simulink model "sensorMCUSlugsMKII_ren"  (Simulink 6.6)
settings: Solver=FixedStepDiscrete  StartTime=0.0  StopTime=10.0  FixedStep=0.01  RelTol=1e-3
InitFcn:
  | mcuInit
values from neighbouring files (symbols this model uses):
  accBiasRateLimit = 2*(.014844)/300*apSampleTime    [mcuInit.m]
  accelXCutTemp = 350.0    (= 350)    [mcuInit.m]
  axTGain1 = -0.0332796    [mcuInit.m]
  axTGain2 = 0.0543519    [mcuInit.m]
  axTMean1 = 68.41    [mcuInit.m]
  axTMean2 = 500.7    [mcuInit.m]
  barAdjust = -6    [mcuInit.m]
  baroCutoff = 0.38/(2*pi)    (= 0.0604788783749)    [mcuInit.m]
  baroCutTemp = -50.0    (= -50)    [mcuInit.m]
  baroOffset = P(2)    [mcuInit.m]
  baroScale = P(1)    [mcuInit.m]
  barTGain1 = -0.0102663    [mcuInit.m]
  barTGain2 = 0.0207608    [mcuInit.m]
  barTMean1 = -161.3    [mcuInit.m]
  barTMean2 = 347.23    [mcuInit.m]
  baseTemp = 288.215    [mcuInit.m]
  cubeAccelGain = (2.522e-3)*9.815    (= 0.02475343)    [mcuInit.m]
  cubeGyroGain = .07326*pi/180    (= 0.00127862821001)    [mcuInit.m]
  gyroBiasRateLimit = 2*(.006393)/500*apSampleTime    [mcuInit.m]
  lapseRate = -0.00198122    [mcuInit.m]
  lowRateSensorCutoff = 0.02    [mcuInit.m]
  magMeanTemp = [162.42 162.42 162.42]    [mcuInit.m]
  magOffset = 0    [mcuInit.m]
  magScale = 0.3418    [mcuInit.m]
  magTempK = [.0057 -.0423 .0426]    [mcuInit.m]
  mainSensorCutoff = 10    [mcuInit.m]
  maxDynPressure = 3000    [mcuInit.m]
  pitAdjust = -41    [mcuInit.m]
  pitCutTemp = -130.0    (= -130)    [mcuInit.m]
  pitotOffset = -1083.881038056753    (= -1083.88103806)    [mcuInit.m]
  pitotScale = 1.213292590242    (= 1.21329259024)    [mcuInit.m]
  pitTGain1 = -0.0552923    [mcuInit.m]
  pitTGain2 = -0.0950433    [mcuInit.m]
  pitTMean1 = -202.93    [mcuInit.m]
  pitTMean2 = 293.053    [mcuInit.m]
  powerOffset = P(2)    [mcuInit.m]
  powerScale = P(1)    [mcuInit.m]
  pressureSensorCutoff = 5    [mcuInit.m]
  T = 0.01    [initGPS.m]    (also in mcuInit.m)
  tempOffset = P(2)    [mcuInit.m]
  tempScale = P(1)    [mcuInit.m]
  vzCutoff = 2    [mcuInit.m]
  xCutoff = 10    [mcuInit.m]
  yCutoff = 10    [mcuInit.m]
  zCutoff = 0.2    [mcuInit.m]
undefined symbols (not defined in the file or in its folder): apSampleTime, baseHeight, DiscIntNeverNeededParam, gaind, getCubeData, getGpsMainData, getMag, GS_location, hil_getEuler, hil_getRates, hil_getRawRead, hil_getVned, hil_getXYZ, hilRead, logData, param_acc, param_mag, polesd, protParseDecode, q_quat, sensorMCUInit, spiSend, u1, u2, updateAirData, updateAttitude, updateBias, updateDiagnosticFl, updateDiagnosticSh, updateLoadData, updatePilotConsole, updatePosition, updateRawADCData, updateTimeStamp, Vb_0, y1, zerosd
libraries: dsPICdrivers x45, simulink x13, aerolibutil x4, dspmtrx3 x2, aerolibconvert2 x2
(part 3 of 4)

== system sensorMCUSlugsMKII_ren/Position and Attitude Filter/Position Filter/BlendPosVel/2 FIlter Blend ==
  HiPass : Inport
  LoPass1 : Inport  Port=2
  1D Filter : Subsystem  AncestorBlock=SLUGS_Library/Singnal Routing & Conditioning/3D Filter  RTWFcnName=TustinFilter3D  mask{zval=[0], pval=-zCutoff, kval=1, TSample=apSampleTime}
      mask prompts: zval "Zeros"; pval "Poles"; kval "Gains"; TSample "Sample Time"
      settings: RTWFcnNameOpts=User specified  RTWFileNameOpts=Use function name
      mask Display:
      | droots(zval,pval,kval)
      | port_label('input',1,'1D')
  Sum : Sum  OutDataTypeMode=single
  "Tustin Lowpass,  Auto Initial Condition4" : Subsystem  mask(Tustin1stOrderLowpassAutoInitialCondition){f=baroCutoff, T=T}
      mask prompts: f "Lowpass Frequency"; T "Sample Time"
      mask help: Takes a 3db rolloff frequency (in Hz, NOT radians/s) and a sample time. Performs a symbolic Tustin conversion and implements in a discrete filter. The initial output of the filter is set by the first sample.
      mask Help: Enter the desired 3db rolloff frequency in Hz and the sample time. Initial conditions are sampled automatically.
      mask Display: fprintf('%.2f Hz lowpass',f)
  Blend : Outport
  wires:
  HiPass/1 -> 1D Filter/1(In1)
  LoPass1/1 -> "Tustin Lowpass,  Auto Initial Condition4"/1(In1)
  1D Filter/1(Out1) -> Sum/1
  "Tustin Lowpass,  Auto Initial Condition4"/1(Out1) -> Sum/2
  Sum/1 -> Blend/1

== system sensorMCUSlugsMKII_ren/Position and Attitude Filter/Position Filter/BlendPosVel/3D Filter ==
  In1 : Inport
  Data Type Conversion1 : DataTypeConversion  OutDataTypeMode=single
  Data Type Conversion2 : DataTypeConversion  OutDataTypeMode=double
  Demux : Demux  Outputs=3
  Filter1 : Subsystem  mask(DiscretizedZeroPole){Zeros=zval, Poles=pval, Gain=kval, AbsTol=auto, SampleTime=TSample, method=tustin, Wc=1}
      mask prompts: Zeros "Zeros (enter in s-main:)"; Poles "Poles (enter in s-domain:)"; Gain "Gain (enter in s-domain:)"; AbsTol "Absolute tolerance:"; SampleTime "Sample time:"; Wc "Critical Frequency (Hz):"
      mask help: Continuous mask uses c2d to transform parameters onto the Discrete Zero-Pole block inside.
      mask init: same as sensorMCUSlugsMKII_ren/Position and Attitude Filter/Attitude Complimentary Filter COG/3D Filter/Filter1
      mask StyleString: edit,edit,edit,edit,edit,popup(zoh|foh|tustin|prewarp|matched),edit
      mask CallbackString: |||||hidecrit|
      mask Display:
      | droots(zeross,poless,gainss)
      | text( 0.5, 1.0, method, 'verticalAlignment','top')
  Filter2 : Subsystem  mask(DiscretizedZeroPole){Zeros=zval, Poles=pval, Gain=kval, AbsTol=auto, SampleTime=TSample, method=tustin, Wc=1}
      mask prompts: Zeros "Zeros (enter in s-main:)"; Poles "Poles (enter in s-domain:)"; Gain "Gain (enter in s-domain:)"; AbsTol "Absolute tolerance:"; SampleTime "Sample time:"; Wc "Critical Frequency (Hz):"
      mask help: Continuous mask uses c2d to transform parameters onto the Discrete Zero-Pole block inside.
      mask init: same as sensorMCUSlugsMKII_ren/Position and Attitude Filter/Attitude Complimentary Filter COG/3D Filter/Filter1
      mask StyleString: edit,edit,edit,edit,edit,popup(zoh|foh|tustin|prewarp|matched),edit
      mask CallbackString: |||||hidecrit|
      mask Display:
      | droots(zeross,poless,gainss)
      | text( 0.5, 1.0, method, 'verticalAlignment','top')
  Filter3 : Subsystem  mask(DiscretizedZeroPole){Zeros=zval, Poles=pval, Gain=kval, AbsTol=auto, SampleTime=TSample, method=tustin, Wc=1}
      mask prompts: Zeros "Zeros (enter in s-main:)"; Poles "Poles (enter in s-domain:)"; Gain "Gain (enter in s-domain:)"; AbsTol "Absolute tolerance:"; SampleTime "Sample time:"; Wc "Critical Frequency (Hz):"
      mask help: Continuous mask uses c2d to transform parameters onto the Discrete Zero-Pole block inside.
      mask init: same as sensorMCUSlugsMKII_ren/Position and Attitude Filter/Attitude Complimentary Filter COG/3D Filter/Filter1
      mask StyleString: edit,edit,edit,edit,edit,popup(zoh|foh|tustin|prewarp|matched),edit
      mask CallbackString: |||||hidecrit|
      mask Display:
      | droots(zeross,poless,gainss)
      | text( 0.5, 1.0, method, 'verticalAlignment','top')
  myMux Fun1 : Stateflow chart
  Out1 : Outport
  wires:
  myMux Fun1/1(y) -> Data Type Conversion1/1
  In1/1 -> Data Type Conversion2/1
  Filter3/1(Out1) -> myMux Fun1/3(u3)
  Filter2/1(Out1) -> myMux Fun1/2(u2)
  Filter1/1(Out1) -> myMux Fun1/1(u1)
  Demux/3 -> Filter3/1(In1)
  Demux/2 -> Filter2/1(In1)
  Demux/1 -> Filter1/1(In1)
  Data Type Conversion2/1 -> Demux/1
  Data Type Conversion1/1 -> Out1/1

== system sensorMCUSlugsMKII_ren/Position and Attitude Filter/Position Filter/BlendPosVel/CompFiltRate ==
  Rate : Inport
  LoPass : Inport  Port=2
  1D Filter1 : Subsystem  AncestorBlock=SLUGS_Library/Singnal Routing & Conditioning/3D Filter  RTWFcnName=TustinFilter3D  mask{zval=[], pval=[0], kval=1, TSample=T}
      mask prompts: zval "Zeros"; pval "Poles"; kval "Gains"; TSample "Sample Time"
      settings: RTWFcnNameOpts=User specified  RTWFileNameOpts=Use function name
      mask Display:
      | droots(zval,pval,kval)
      | port_label('input',1,'1D')
  Gain : Gain  Gain=omega
  Sum : Sum  Inputs=++|
  Sum1 : Sum  Inputs=|+-
  Unit Delay : UnitDelay  Orientation=left  SampleTime=T
  Blend : Outport
  wires:
  Unit Delay/1 -> Sum1/2
  LoPass/1 -> Sum1/1
  Sum1/1 -> Gain/1
  Gain/1 -> Sum/2
  Rate/1 -> Sum/1
  Sum/1 -> 1D Filter1/1(In1)
  1D Filter1/1(Out1) -> Unit Delay/1, Blend/1

== system sensorMCUSlugsMKII_ren/Position and Attitude Filter/Position Filter/BlendPosVel/CompFiltRate1 ==
  Rate : Inport
  LoPass : Inport  Port=2
  1D Filter1 : Subsystem  AncestorBlock=SLUGS_Library/Singnal Routing & Conditioning/3D Filter  RTWFcnName=TustinFilter3D  mask{zval=[], pval=[0], kval=1, TSample=T}
      mask prompts: zval "Zeros"; pval "Poles"; kval "Gains"; TSample "Sample Time"
      settings: RTWFcnNameOpts=User specified  RTWFileNameOpts=Use function name
      mask Display:
      | droots(zval,pval,kval)
      | port_label('input',1,'1D')
  Gain : Gain  Gain=omega
  Sum : Sum  Inputs=++|
  Sum1 : Sum  Inputs=|+-
  Unit Delay : UnitDelay  Orientation=left  SampleTime=T
  Blend : Outport
  wires:
  Unit Delay/1 -> Sum1/2
  LoPass/1 -> Sum1/1
  Sum1/1 -> Gain/1
  Gain/1 -> Sum/2
  Rate/1 -> Sum/1
  Sum/1 -> 1D Filter1/1(In1)
  1D Filter1/1(Out1) -> Unit Delay/1, Blend/1

== system sensorMCUSlugsMKII_ren/Position and Attitude Filter/Position Filter/BlendPosVel/CompRateOnly ==
  LoPass : Inport
  1D Filter1 : Subsystem  AncestorBlock=SLUGS_Library/Singnal Routing & Conditioning/3D Filter  RTWFcnName=TustinFilter3D  mask{zval=[], pval=[0], kval=1, TSample=T}
      mask prompts: zval "Zeros"; pval "Poles"; kval "Gains"; TSample "Sample Time"
      settings: RTWFcnNameOpts=User specified  RTWFileNameOpts=Use function name
      mask Display:
      | droots(zval,pval,kval)
      | port_label('input',1,'1D')
  Gain : Gain  Gain=omega
  Sum1 : Sum  Inputs=|+-
  Unit Delay : UnitDelay  Orientation=left  SampleTime=T
  Rate_hat : Outport
  wires:
  Unit Delay/1 -> Sum1/2
  LoPass/1 -> Sum1/1
  Sum1/1 -> Gain/1
  Gain/1 -> Rate_hat/1, 1D Filter1/1(In1)
  1D Filter1/1(Out1) -> Unit Delay/1

== system sensorMCUSlugsMKII_ren/Position and Attitude Filter/Position Filter/BlendPosVel/Subsystem ==
  Vn : Inport
  Ve : Inport  Port=2
  New GPS : Inport  Orientation=up  Port=3
  Enable : EnablePort
  Embedded MATLAB Function : Stateflow chart
  Embedded MATLAB Function1 : Stateflow chart
  Vn_fil : Outport  OutputWhenDisabled=reset  InitialOutput=0
  Ve_fil : Outport  Port=2  OutputWhenDisabled=reset  InitialOutput=0
  wires:
  New GPS/1 -> Embedded MATLAB Function1/2(NewGPS), Embedded MATLAB Function/2(NewGPS)
  Vn/1 -> Embedded MATLAB Function/1(u)
  Ve/1 -> Embedded MATLAB Function1/1(u)
  Embedded MATLAB Function/1(y) -> Vn_fil/1
  Embedded MATLAB Function1/1(y) -> Ve_fil/1

== system sensorMCUSlugsMKII_ren/Sensor Data/Sensor Suite/Cube Signal Cond1/3D Tustin Lowpass, Auto Initial Condition ==
  In1 : Inport
  Constant : Constant  Value=T
  Constant1 : Constant  Value=f
  Constant2 : Constant  Value=T
  Constant3 : Constant  Value=f
  Constant4 : Constant  Value=T
  Constant5 : Constant  Value=f
  Demux : Demux  Outputs=3
  Embedded MATLAB Function : Stateflow chart
  Embedded MATLAB Function1 : Stateflow chart
  Embedded MATLAB Function2 : Stateflow chart
  myMux Fun : Stateflow chart
  Out1 : Outport
  wires:
  myMux Fun/1(y) -> Out1/1
  In1/1 -> Demux/1
  Embedded MATLAB Function1/1(y) -> myMux Fun/2(u2)
  Demux/3 -> Embedded MATLAB Function2/1(u)
  Demux/2 -> Embedded MATLAB Function1/1(u)
  Demux/1 -> Embedded MATLAB Function/1(u)
  Embedded MATLAB Function2/1(y) -> myMux Fun/3(u3)
  Constant5/1 -> Embedded MATLAB Function2/3(f)
  Constant4/1 -> Embedded MATLAB Function2/2(T)
  Constant3/1 -> Embedded MATLAB Function1/3(f)
  Constant2/1 -> Embedded MATLAB Function1/2(T)
  Embedded MATLAB Function/1(y) -> myMux Fun/1(u1)
  Constant1/1 -> Embedded MATLAB Function/3(f)
  Constant/1 -> Embedded MATLAB Function/2(T)

== system sensorMCUSlugsMKII_ren/Sensor Data/Sensor Suite/Cube Signal Cond1/3D Tustin Lowpass, Auto Initial Condition1 ==
  In1 : Inport
  Constant : Constant  Value=T
  Constant1 : Constant  Value=f
  Constant2 : Constant  Value=T
  Constant3 : Constant  Value=f
  Constant4 : Constant  Value=T
  Constant5 : Constant  Value=f
  Demux : Demux  Outputs=3
  Embedded MATLAB Function : Stateflow chart
  Embedded MATLAB Function1 : Stateflow chart
  Embedded MATLAB Function2 : Stateflow chart
  myMux Fun : Stateflow chart
  Out1 : Outport
  wires:
  myMux Fun/1(y) -> Out1/1
  In1/1 -> Demux/1
  Embedded MATLAB Function1/1(y) -> myMux Fun/2(u2)
  Demux/3 -> Embedded MATLAB Function2/1(u)
  Demux/2 -> Embedded MATLAB Function1/1(u)
  Demux/1 -> Embedded MATLAB Function/1(u)
  Embedded MATLAB Function2/1(y) -> myMux Fun/3(u3)
  Constant5/1 -> Embedded MATLAB Function2/3(f)
  Constant4/1 -> Embedded MATLAB Function2/2(T)
  Constant3/1 -> Embedded MATLAB Function1/3(f)
  Constant2/1 -> Embedded MATLAB Function1/2(T)
  Embedded MATLAB Function/1(y) -> myMux Fun/1(u1)
  Constant1/1 -> Embedded MATLAB Function/3(f)
  Constant/1 -> Embedded MATLAB Function/2(T)

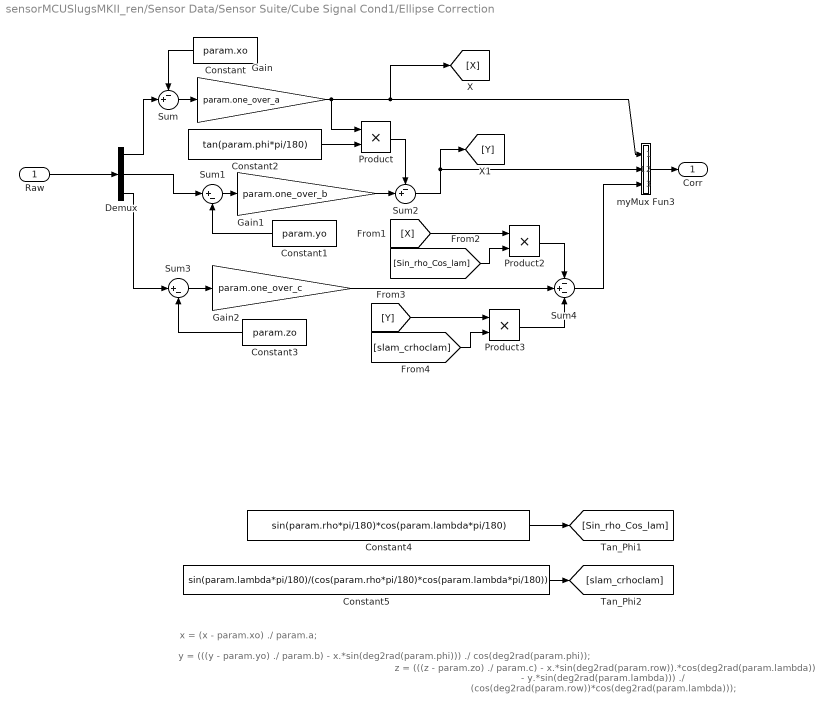
== system sensorMCUSlugsMKII_ren/Sensor Data/Sensor Suite/Cube Signal Cond1/Ellipse Correction ==
  note: x = (x - param.xo) ./ param.a;
  note: y = (((y - param.yo) ./ param.b) - x.*sin(deg2rad(param.phi))) ./ cos(deg2rad(param.phi));
  note: z = (((z - param.zo) ./ param.c) - x.*sin(deg2rad(param.row)).*cos(deg2rad(param.lambda)) - y.*sin(deg2rad(param.lambda))) ./ (cos(deg2rad(param.row))*cos(deg2rad(param.lambda)));
  Raw : Inport
  Constant : Constant  Orientation=left  Value=param.xo  OutDataTypeMode=single
  Constant1 : Constant  Orientation=left  Value=param.yo  OutDataTypeMode=single
  Constant2 : Constant  Value=tan(param.phi*pi/180)  OutDataTypeMode=single
  Constant3 : Constant  Orientation=left  Value=param.zo  OutDataTypeMode=single
  Constant4 : Constant  Value=sin(param.rho*pi/180)*cos(param.lambda*pi/180)  OutDataTypeMode=single
  Constant5 : Constant  Value=sin(param.lambda*pi/180)/(cos(param.rho*pi/180)*cos(param.lambda*pi/180))  VectorParams1D=off  OutDataTypeMode=single
  Demux : Demux  Outputs=3
  Gain : Gain  Gain=param.one_over_a
  Gain1 : Gain  Gain=param.one_over_b
  Gain2 : Gain  Gain=param.one_over_c
  Product : Product  RndMeth=Zero
  Product2 : Product  RndMeth=Zero
  Product3 : Product  RndMeth=Zero
  Sum : Sum  Inputs=-+|
  Sum1 : Sum  Inputs=|+-
  Sum2 : Sum  Inputs=-+|
  Sum3 : Sum  Inputs=|+-
  Sum4 : Sum  Inputs=-+-
  myMux Fun3 : Stateflow chart  AncestorBlock=SLUGS_Library/Singnal Routing & Conditioning/myMux Fun3
  Corr : Outport
  wires:
  Raw/1 -> Demux/1
  Demux/1 -> Sum/2
  Constant/1 -> Sum/1
  Sum/1 -> Gain/1
  Gain/1 -> [X], Product/1, myMux Fun3/1(u1)
  Sum1/1 -> Gain1/1
  myMux Fun3/1(y) -> Corr/1
  Constant1/1 -> Sum1/2
  Demux/2 -> Sum1/1
  Constant2/1 -> Product/2
  Gain1/1 -> Sum2/2
  Product/1 -> Sum2/1
  Sum2/1 -> [Y], myMux Fun3/2(u2)
  Sum3/1 -> Gain2/1
  Constant3/1 -> Sum3/2
  Gain2/1 -> Sum4/2
  Demux/3 -> Sum3/1
  [X] -> Product2/1
  [Sin_rho_Cos_lam] -> Product2/2
  Product2/1 -> Sum4/1
  [Y] -> Product3/1
  [slam_crhoclam] -> Product3/2
  Product3/1 -> Sum4/3
  Sum4/1 -> myMux Fun3/3(u3)
  Constant4/1 -> [Sin_rho_Cos_lam]
  Constant5/1 -> [slam_crhoclam]

== system sensorMCUSlugsMKII_ren/Sensor Data/Sensor Suite/Cube Signal Cond1/Rotate Cube Axis ==
  Raw : Inport
  Selector : Selector  IndexOptions=Index vector (dialog)  Indices=[2 1 3]  OutputSizes=1  InputPortWidth=3
  "[ -1 -1 -1]" : Gain  Gain=[-1 -1 -1]
  Rotated : Outport
  wires:
  Selector/1 -> "[ -1 -1 -1]"/1
  Raw/1 -> Selector/1
  "[ -1 -1 -1]"/1 -> Rotated/1

== system sensorMCUSlugsMKII_ren/Sensor Data/Sensor Suite/Cube Signal Cond1/Rotate Cube Axis  ==
  Raw : Inport
  Selector : Selector  IndexOptions=Index vector (dialog)  Indices=[2 1 3]  OutputSizes=1  InputPortWidth=3
  Rotated : Outport
  wires:
  Raw/1 -> Selector/1
  Selector/1 -> Rotated/1

== system sensorMCUSlugsMKII_ren/Sensor Data/Sensor Suite/Cube Signal Cond1/Temp Compensate Accel X ==
  Temp : Inport
  Accel X : Inport  Port=2
  Compare To Constant : simulink/Logic and Bit Operations/Compare To Constant  SystemSampleTime=-1  relop=<  const=accelXCutTemp  LogicOutDataTypeMode=uint8  ZeroCross=off
  Hi Temp Compensation : Subsystem  mask{alpha=axTGain2, tempMean=axTMean2}
      mask prompts: alpha "Tempearature Coeficient (K_t)"; tempMean "Calibration Temperature Mean (T_avg)"
      mask help:
      | This block implements a temperature compensation. It implmements the following equation:
      |
      | M_tc = M_raw - K_t(T - T_avg)
  Lo Temp Compensation : Subsystem  mask{alpha=axTGain1, tempMean=axTMean1}
      mask prompts: alpha "Tempearature Coeficient (K_t)"; tempMean "Calibration Temperature Mean (T_avg)"
      mask help:
      | This block implements a temperature compensation. It implmements the following equation:
      |
      | M_tc = M_raw - K_t(T - T_avg)
  Logical Operator : Logic  Operator=NOT  AllPortsSameDT=off  OutDataTypeMode=Boolean
  Merge : Merge
  "Tustin Lowpass, Auto Initial Condition1" : Subsystem  mask(Tustin1stOrderLowpassAutoInitialCondition){f=1, T=T}
      mask prompts: f "Lowpass Frequency"; T "Sample Time"
      mask help: Takes a 3db rolloff frequency (in Hz, NOT radians/s) and a sample time. Performs a symbolic Tustin conversion and implements in a discrete filter. The initial output of the filter is set by the first sample.
      mask Help: Enter the desired 3db rolloff frequency in Hz and the sample time. Initial conditions are sampled automatically.
      mask Display: fprintf('%.2f Hz lowpass',f)
  Accel X_c : Outport
  wires:
  "Tustin Lowpass, Auto Initial Condition1"/1(Out1) -> Accel X_c/1
  Compare To Constant/1 -> Logical Operator/1, Lo Temp Compensation/Enable
  Temp/1 -> Compare To Constant/1, Hi Temp Compensation/2(Temp Raw), Lo Temp Compensation/2(Temp Raw)
  Accel X/1 -> Hi Temp Compensation/1(Raw), Lo Temp Compensation/1(Raw)
  Hi Temp Compensation/1(Comp) -> Merge/1
  Lo Temp Compensation/1(Comp) -> Merge/2
  Merge/1 -> "Tustin Lowpass, Auto Initial Condition1"/1(In1)
  Logical Operator/1 -> Hi Temp Compensation/Enable

== system sensorMCUSlugsMKII_ren/Sensor Data/Sensor Suite/Low Pass Filtering,Temperature Compensation and Calibration1/3D Tustin Lowpass, Auto Initial Condition ==
  In1 : Inport
  Constant : Constant  Value=T
  Constant1 : Constant  Value=f
  Constant2 : Constant  Value=T
  Constant3 : Constant  Value=f
  Constant4 : Constant  Value=T
  Constant5 : Constant  Value=f
  Demux : Demux  Outputs=3
  Embedded MATLAB Function : Stateflow chart
  Embedded MATLAB Function1 : Stateflow chart
  Embedded MATLAB Function2 : Stateflow chart
  myMux Fun : Stateflow chart
  Out1 : Outport
  wires:
  myMux Fun/1(y) -> Out1/1
  In1/1 -> Demux/1
  Embedded MATLAB Function1/1(y) -> myMux Fun/2(u2)
  Demux/3 -> Embedded MATLAB Function2/1(u)
  Demux/2 -> Embedded MATLAB Function1/1(u)
  Demux/1 -> Embedded MATLAB Function/1(u)
  Embedded MATLAB Function2/1(y) -> myMux Fun/3(u3)
  Constant5/1 -> Embedded MATLAB Function2/3(f)
  Constant4/1 -> Embedded MATLAB Function2/2(T)
  Constant3/1 -> Embedded MATLAB Function1/3(f)
  Constant2/1 -> Embedded MATLAB Function1/2(T)
  Embedded MATLAB Function/1(y) -> myMux Fun/1(u1)
  Constant1/1 -> Embedded MATLAB Function/3(f)
  Constant/1 -> Embedded MATLAB Function/2(T)

== system sensorMCUSlugsMKII_ren/Sensor Data/Sensor Suite/Low Pass Filtering,Temperature Compensation and Calibration1/Baro Altimeter ==
  Static (Pa) : Inport  Orientation=up
  Compute Barometric Height : Subsystem  mask{baseTemp=baseTemp, LapseRate=lapseRate}
      mask prompts: baseTemp "Base Station Temperature (K)"; LapseRate "Lapse Rate (C/ft)"
      mask help:
      | Produces Altitude in meters from Barometric Pressure in Pascals. Altitude is valid from MSL to 6000 ft.
      |
      | The method implemented here was developed by Ren Curry
  Constant1 : Constant  Value=baseHeight  OutDataTypeMode=single
  Enabled Subsystem : Subsystem  TreatAsAtomicUnit=on
  Enables/Disables the Computation of  initial Baro Bias : Stateflow chart
  Initial Baro Bias : Subsystem  TreatAsAtomicUnit=on
  Logical Operator : Logic  Orientation=down  Operator=NOT  AllPortsSameDT=off  OutDataTypeMode=Boolean
  Sum1 : Sum  Inputs=++|  OutDataTypeMode=single
  Zero Out Height : Subsystem  TreatAsAtomicUnit=on
  Altitude : Outport
  wires:
  Compute Barometric Height/1("Altitude, m") -> Zero Out Height/2(Computed Height), Sum1/2
  Static (Pa)/1 -> Initial Baro Bias/1(Baro (Pa)), Compute Barometric Height/3(Baro (Pa))
  Enables/Disables the Computation of  initial Baro Bias/1(tOut) -> Initial Baro Bias/Enable, Zero Out Height/Enable, Logical Operator/1
  Constant1/1 -> Compute Barometric Height/1(Base Height (m)), Zero Out Height/1(Base Height)
  Initial Baro Bias/1(Baro (Gnd)) -> Compute Barometric Height/2(Base Pressure (Pa))
  Zero Out Height/1(Height Offset) -> Sum1/1
  Logical Operator/1 -> Enabled Subsystem/Enable
  Sum1/1 -> Enabled Subsystem/1(In1)
  Enabled Subsystem/1(Out1) -> Altitude/1

== system sensorMCUSlugsMKII_ren/Sensor Data/Sensor Suite/Low Pass Filtering,Temperature Compensation and Calibration1/Barometer Unit Conversion ==
  Raw : Inport
  Bias : Constant  Value=bias  OutDataTypeMode=single
  Divide : Product  OutDataTypeMode=single  OutScaling=2^-10
  Gains : Constant  Value=gains  OutDataTypeMode=single
  Sum : Sum  Inputs=|++  OutDataTypeMode=single
  Comp : Outport
  wires:
  Bias/1 -> Sum/2
  Raw/1 -> Divide/2
  Gains/1 -> Divide/1
  Divide/1 -> Sum/1
  Sum/1 -> Comp/1

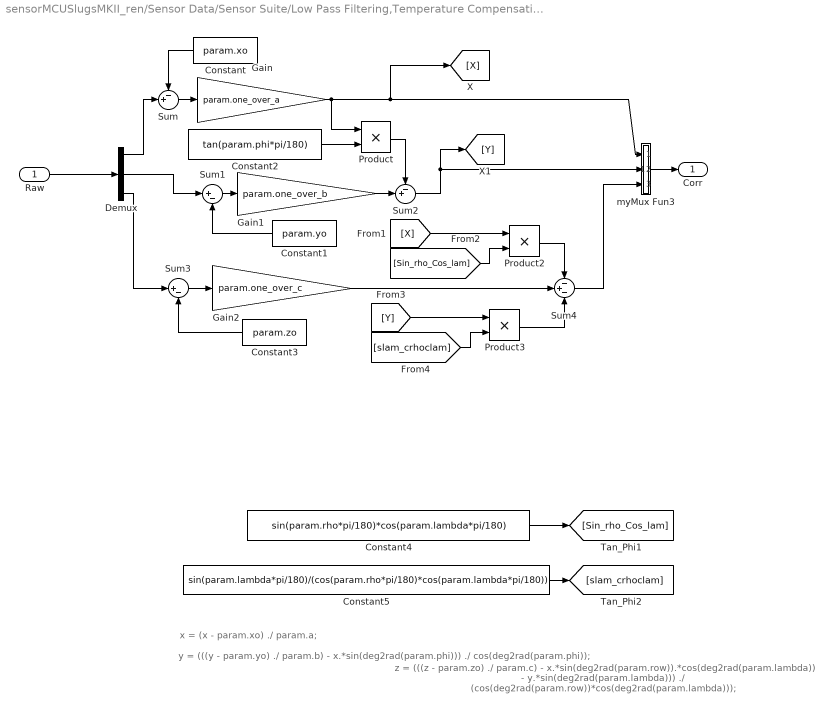
== system sensorMCUSlugsMKII_ren/Sensor Data/Sensor Suite/Low Pass Filtering,Temperature Compensation and Calibration1/Ellipse Correction ==
  note: x = (x - param.xo) ./ param.a;
  note: y = (((y - param.yo) ./ param.b) - x.*sin(deg2rad(param.phi))) ./ cos(deg2rad(param.phi));
  note: z = (((z - param.zo) ./ param.c) - x.*sin(deg2rad(param.row)).*cos(deg2rad(param.lambda)) - y.*sin(deg2rad(param.lambda))) ./ (cos(deg2rad(param.row))*cos(deg2rad(param.lambda)));
  Raw : Inport
  Constant : Constant  Orientation=left  Value=param.xo  OutDataTypeMode=single
  Constant1 : Constant  Orientation=left  Value=param.yo  OutDataTypeMode=single
  Constant2 : Constant  Value=tan(param.phi*pi/180)  OutDataTypeMode=single
  Constant3 : Constant  Orientation=left  Value=param.zo  OutDataTypeMode=single
  Constant4 : Constant  Value=sin(param.rho*pi/180)*cos(param.lambda*pi/180)  OutDataTypeMode=single
  Constant5 : Constant  Value=sin(param.lambda*pi/180)/(cos(param.rho*pi/180)*cos(param.lambda*pi/180))  VectorParams1D=off  OutDataTypeMode=single
  Demux : Demux  Outputs=3
  Gain : Gain  Gain=param.one_over_a
  Gain1 : Gain  Gain=param.one_over_b
  Gain2 : Gain  Gain=param.one_over_c
  Product : Product  RndMeth=Zero
  Product2 : Product  RndMeth=Zero
  Product3 : Product  RndMeth=Zero
  Sum : Sum  Inputs=-+|
  Sum1 : Sum  Inputs=|+-
  Sum2 : Sum  Inputs=-+|
  Sum3 : Sum  Inputs=|+-
  Sum4 : Sum  Inputs=-+-
  myMux Fun3 : Stateflow chart  AncestorBlock=SLUGS_Library/Singnal Routing & Conditioning/myMux Fun3
  Corr : Outport
  wires:
  Raw/1 -> Demux/1
  Demux/1 -> Sum/2
  Constant/1 -> Sum/1
  Sum/1 -> Gain/1
  Gain/1 -> [X], Product/1, myMux Fun3/1(u1)
  Sum1/1 -> Gain1/1
  myMux Fun3/1(y) -> Corr/1
  Constant1/1 -> Sum1/2
  Demux/2 -> Sum1/1
  Constant2/1 -> Product/2
  Gain1/1 -> Sum2/2
  Product/1 -> Sum2/1
  Sum2/1 -> [Y], myMux Fun3/2(u2)
  Sum3/1 -> Gain2/1
  Constant3/1 -> Sum3/2
  Gain2/1 -> Sum4/2
  Demux/3 -> Sum3/1
  [X] -> Product2/1
  [Sin_rho_Cos_lam] -> Product2/2
  Product2/1 -> Sum4/1
  [Y] -> Product3/1
  [slam_crhoclam] -> Product3/2
  Product3/1 -> Sum4/3
  Sum4/1 -> myMux Fun3/3(u3)
  Constant4/1 -> [Sin_rho_Cos_lam]
  Constant5/1 -> [slam_crhoclam]

== system sensorMCUSlugsMKII_ren/Sensor Data/Sensor Suite/Low Pass Filtering,Temperature Compensation and Calibration1/Magnetometer Unit Conversion ==
  Raw : Inport
  Bias : Constant  Value=bias  OutDataTypeMode=single
  Divide : Product  OutDataTypeMode=single  OutScaling=2^-10
  Gains : Constant  Value=gains  OutDataTypeMode=single
  Sum : Sum  Inputs=|++  OutDataTypeMode=single
  Comp : Outport
  wires:
  Bias/1 -> Sum/2
  Raw/1 -> Divide/2
  Gains/1 -> Divide/1
  Divide/1 -> Sum/1
  Sum/1 -> Comp/1

== system sensorMCUSlugsMKII_ren/Sensor Data/Sensor Suite/Low Pass Filtering,Temperature Compensation and Calibration1/Magnetometers Temp Compensation ==
  Raw : Inport
  Temp Raw : Inport  Port=2
  Divide1 : Product  OutDataTypeMode=single  OutScaling=2^-10
  Mean Temperature for Calibration : Constant  Value=tempMean  OutDataTypeMode=single
  Sum1 : Sum  Inputs=|+-  OutDataTypeMode=single
  Sum2 : Sum  Inputs=|+-  OutDataTypeMode=single
  gains : Constant  Value=alpha  OutDataTypeMode=single
  Comp : Outport
  wires:
  Sum2/1 -> Comp/1
  Divide1/1 -> Sum2/2
  gains/1 -> Divide1/1
  Sum1/1 -> Divide1/2
  Temp Raw/1 -> Sum1/1
  Raw/1 -> Sum2/1
  Mean Temperature for Calibration/1 -> Sum1/2

== system sensorMCUSlugsMKII_ren/Sensor Data/Sensor Suite/Low Pass Filtering,Temperature Compensation and Calibration1/Pitot Unit Conversion ==
  Raw : Inport
  Bias : Constant  Value=bias  OutDataTypeMode=single
  Divide : Product  OutDataTypeMode=single  OutScaling=2^-10
  Gains : Constant  Value=gains  OutDataTypeMode=single
  Sum : Sum  Inputs=|++  OutDataTypeMode=single
  Comp : Outport
  wires:
  Bias/1 -> Sum/2
  Raw/1 -> Divide/2
  Gains/1 -> Divide/1
  Divide/1 -> Sum/1
  Sum/1 -> Comp/1

== system sensorMCUSlugsMKII_ren/Sensor Data/Sensor Suite/Low Pass Filtering,Temperature Compensation and Calibration1/Power Unit Conversion ==
  Raw : Inport
  Bias : Constant  Value=bias  OutDataTypeMode=single
  Divide : Product  OutDataTypeMode=single  OutScaling=2^-10
  Gains : Constant  Value=gains  OutDataTypeMode=single
  Sum : Sum  Inputs=|++  OutDataTypeMode=single
  Comp : Outport
  wires:
  Bias/1 -> Sum/2
  Raw/1 -> Divide/2
  Gains/1 -> Divide/1
  Divide/1 -> Sum/1
  Sum/1 -> Comp/1

== system sensorMCUSlugsMKII_ren/Sensor Data/Sensor Suite/Low Pass Filtering,Temperature Compensation and Calibration1/Rotate Mags Axis ==
  Raw : Inport
  Selector : Selector  IndexOptions=Index vector (dialog)  Indices=[2 1 3]  OutputSizes=1  InputPortWidth=3
  "[ 1 -1 1]" : Gain  Gain=[-1 -1 1]
  Rotated : Outport
  wires:
  Selector/1 -> "[ 1 -1 1]"/1
  Raw/1 -> Selector/1
  "[ 1 -1 1]"/1 -> Rotated/1

== system sensorMCUSlugsMKII_ren/Sensor Data/Sensor Suite/Low Pass Filtering,Temperature Compensation and Calibration1/Temp Compensate Accel X1 ==
  Temp : Inport
  Dynamic : Inport  Port=2
  Compare To Constant : simulink/Logic and Bit Operations/Compare To Constant  SystemSampleTime=-1  relop=<  const=pitCutTemp  LogicOutDataTypeMode=uint8  ZeroCross=off
  Display : Display
  Display2 : Display
  Hi Temp Compensation2 : Subsystem  mask{alpha=pitTGain2, tempMean=pitTMean2}
      mask prompts: alpha "Tempearature Coeficient (K_t)"; tempMean "Calibration Temperature Mean (T_avg)"
      mask help:
      | This block implements a temperature compensation. It implmements the following equation:
      |
      | M_tc = M_raw - K_t(T - T_avg)
  Lo Temp Compensation : Subsystem  mask{alpha=pitTGain1, tempMean=pitTMean1}
      mask prompts: alpha "Tempearature Coeficient (K_t)"; tempMean "Calibration Temperature Mean (T_avg)"
      mask help:
      | This block implements a temperature compensation. It implmements the following equation:
      |
      | M_tc = M_raw - K_t(T - T_avg)
  Logical Operator : Logic  Operator=NOT  AllPortsSameDT=off  OutDataTypeMode=Boolean
  Merge : Merge
  Baro_c : Outport
  wires:
  Hi Temp Compensation2/1(Comp) -> Merge/1
  Logical Operator/1 -> Hi Temp Compensation2/Enable, Display2/1
  Merge/1 -> Baro_c/1, Display/1
  Dynamic/1 -> Lo Temp Compensation/1(Raw), Hi Temp Compensation2/1(Raw)
  Temp/1 -> Compare To Constant/1, Lo Temp Compensation/2(Temp Raw), Hi Temp Compensation2/2(Temp Raw)
  Compare To Constant/1 -> Lo Temp Compensation/Enable, Logical Operator/1
  Lo Temp Compensation/1(Comp) -> Merge/2

== system sensorMCUSlugsMKII_ren/Sensor Data/Sensor Suite/Low Pass Filtering,Temperature Compensation and Calibration1/Temp Compensate Baro ==
  Temp : Inport
  Baro : Inport  Port=2
  Compare To Constant : simulink/Logic and Bit Operations/Compare To Constant  SystemSampleTime=-1  relop=<  const=baroCutTemp  LogicOutDataTypeMode=uint8  ZeroCross=off
  Hi Temp Compensation : Subsystem  mask{alpha=barTGain2, tempMean=barTMean2}
      mask prompts: alpha "Tempearature Coeficient (K_t)"; tempMean "Calibration Temperature Mean (T_avg)"
      mask help:
      | This block implements a temperature compensation. It implmements the following equation:
      |
      | M_tc = M_raw - K_t(T - T_avg)
  Lo Temp Compensation : Subsystem  mask{alpha=barTGain1, tempMean=barTMean1}
      mask prompts: alpha "Tempearature Coeficient (K_t)"; tempMean "Calibration Temperature Mean (T_avg)"
      mask help:
      | This block implements a temperature compensation. It implmements the following equation:
      |
      | M_tc = M_raw - K_t(T - T_avg)
  Logical Operator : Logic  Operator=NOT  AllPortsSameDT=off  OutDataTypeMode=Boolean
  Merge : Merge
  Baro_c : Outport
  wires:
  Compare To Constant/1 -> Logical Operator/1, Lo Temp Compensation/Enable
  Temp/1 -> Compare To Constant/1, Hi Temp Compensation/2(Temp Raw), Lo Temp Compensation/2(Temp Raw)
  Baro/1 -> Hi Temp Compensation/1(Raw), Lo Temp Compensation/1(Raw)
  Lo Temp Compensation/1(Comp) -> Merge/2
  Merge/1 -> Baro_c/1
  Logical Operator/1 -> Hi Temp Compensation/Enable
  Hi Temp Compensation/1(Comp) -> Merge/1

== system sensorMCUSlugsMKII_ren/Sensor Data/Sensor Suite/Low Pass Filtering,Temperature Compensation and Calibration1/Thermistor Unit Conversion ==
  Raw : Inport
  Bias : Constant  Value=bias  OutDataTypeMode=single
  Divide : Product  OutDataTypeMode=single  OutScaling=2^-10
  Gains : Constant  Value=gains  OutDataTypeMode=single
  Sum : Sum  Inputs=|++  OutDataTypeMode=single
  Comp : Outport
  wires:
  Sum/1 -> Comp/1
  Divide/1 -> Sum/1
  Gains/1 -> Divide/1
  Raw/1 -> Divide/2
  Bias/1 -> Sum/2

== system sensorMCUSlugsMKII_ren/Sensor Data/Sensor Suite/Low Pass Filtering,Temperature Compensation and Calibration1/Tustin Lowpass, Auto Initial Condition1 ==
  In1 : Inport
  Constant : Constant  Value=T
  Constant1 : Constant  Value=f
  Embedded MATLAB Function : Stateflow chart
  Out1 : Outport
  wires:
  Constant/1 -> Embedded MATLAB Function/2(T)
  Constant1/1 -> Embedded MATLAB Function/3(f)
  Embedded MATLAB Function/1(y) -> Out1/1
  In1/1 -> Embedded MATLAB Function/1(u)

== system sensorMCUSlugsMKII_ren/Sensor Data/Sensor Suite/Low Pass Filtering,Temperature Compensation and Calibration1/Tustin Lowpass, Auto Initial Condition2 ==
  In1 : Inport
  Constant : Constant  Value=T
  Constant1 : Constant  Value=f
  Embedded MATLAB Function : Stateflow chart
  Out1 : Outport
  wires:
  In1/1 -> Embedded MATLAB Function/1(u)
  Embedded MATLAB Function/1(y) -> Out1/1
  Constant1/1 -> Embedded MATLAB Function/3(f)
  Constant/1 -> Embedded MATLAB Function/2(T)

== system sensorMCUSlugsMKII_ren/Sensor Data/Sensor Suite/Low Pass Filtering,Temperature Compensation and Calibration1/Tustin Lowpass, Auto Initial Condition3 ==
  In1 : Inport
  Constant : Constant  Value=T
  Constant1 : Constant  Value=f
  Embedded MATLAB Function : Stateflow chart
  Out1 : Outport
  wires:
  Constant/1 -> Embedded MATLAB Function/2(T)
  Constant1/1 -> Embedded MATLAB Function/3(f)
  Embedded MATLAB Function/1(y) -> Out1/1
  In1/1 -> Embedded MATLAB Function/1(u)

== system sensorMCUSlugsMKII_ren/Sensor Data/Sensor Suite/Low Pass Filtering,Temperature Compensation and Calibration1/Tustin Lowpass, Auto Initial Condition4 ==
  In1 : Inport
  Constant : Constant  Value=T
  Constant1 : Constant  Value=f
  Embedded MATLAB Function : Stateflow chart
  Out1 : Outport
  wires:
  In1/1 -> Embedded MATLAB Function/1(u)
  Embedded MATLAB Function/1(y) -> Out1/1
  Constant1/1 -> Embedded MATLAB Function/3(f)
  Constant/1 -> Embedded MATLAB Function/2(T)

== system sensorMCUSlugsMKII_ren/Sensor Data/Sensor Suite/Low Pass Filtering,Temperature Compensation and Calibration1/ValidateMags ==
  In1 : Inport
  Hold if Outlier : Subsystem  TreatAsAtomicUnit=on
  Monitor Norm : Subsystem
  Out1 : Outport
  wires:
  In1/1 -> Monitor Norm/1(Mags), Hold if Outlier/1(In1)
  Monitor Norm/1(Enable) -> Hold if Outlier/Enable
  Hold if Outlier/1(Out1) -> Out1/1

== system sensorMCUSlugsMKII_ren/Position and Attitude Filter/Attitude Complimentary Filter COG/Normalize Vector1/Norm/Subsystem2 ==
  x : Inport
  C Function Call : dsPICdrivers/OTHERS/C Function Call  Tag=dsPIC_dsPIC_CFunctionCall  fctName='mySqrt'  INPUT_SIZE=1  INPUT1=real32  INPUT2=--  INPUT3=--  OUTPUT_SIZE=1  OUTPUT1=real32  SampleTime=-1  InputType=[ 7 ]  OutputType=[ 7 ]  FctDeclaration=extern real32_T mySqrt(real32_T u1);  FctCall=%y1 = mySqrt(%u1);  OrderingInOutPopup=None
  negprotect : Stateflow chart
  sqrt(x) : Outport
  wires:
  negprotect/1(zpVal) -> C Function Call/1
  x/1 -> negprotect/1(val)
  C Function Call/1 -> sqrt(x)/1

== system sensorMCUSlugsMKII_ren/Position and Attitude Filter/Attitude Complimentary Filter COG/Normalize Vector1/Norm/Subsystem3 ==
  x : Inport
  y : Inport  Port=2
  Embedded MATLAB Function : Stateflow chart
  x dot y : Outport
  wires:
  y/1 -> Embedded MATLAB Function/2(y)
  x/1 -> Embedded MATLAB Function/1(x)
  Embedded MATLAB Function/1(xDoty) -> x dot y/1

== system sensorMCUSlugsMKII_ren/Position and Attitude Filter/Attitude Complimentary Filter COG/Normalize Vector2/Norm/Subsystem2 ==
  x : Inport
  C Function Call : dsPICdrivers/OTHERS/C Function Call  Tag=dsPIC_dsPIC_CFunctionCall  fctName='mySqrt'  INPUT_SIZE=1  INPUT1=real32  INPUT2=--  INPUT3=--  OUTPUT_SIZE=1  OUTPUT1=real32  SampleTime=-1  InputType=[ 7 ]  OutputType=[ 7 ]  FctDeclaration=extern real32_T mySqrt(real32_T u1);  FctCall=%y1 = mySqrt(%u1);  OrderingInOutPopup=None
  negprotect : Stateflow chart
  sqrt(x) : Outport
  wires:
  C Function Call/1 -> sqrt(x)/1
  x/1 -> negprotect/1(val)
  negprotect/1(zpVal) -> C Function Call/1

== system sensorMCUSlugsMKII_ren/Position and Attitude Filter/Attitude Complimentary Filter COG/Normalize Vector2/Norm/Subsystem3 ==
  x : Inport
  y : Inport  Port=2
  Embedded MATLAB Function : Stateflow chart
  x dot y : Outport
  wires:
  Embedded MATLAB Function/1(xDoty) -> x dot y/1
  x/1 -> Embedded MATLAB Function/1(x)
  y/1 -> Embedded MATLAB Function/2(y)

== system sensorMCUSlugsMKII_ren/Position and Attitude Filter/Attitude Complimentary Filter COG/Quaternion Normalize/Quaternion Modulus/Subsystem1 ==
  x : Inport
  C Function Call : dsPICdrivers/OTHERS/C Function Call  Tag=dsPIC_dsPIC_CFunctionCall  fctName='mySqrt'  INPUT_SIZE=1  INPUT1=real32  INPUT2=--  INPUT3=--  OUTPUT_SIZE=1  OUTPUT1=real32  SampleTime=-1  InputType=[ 7 ]  OutputType=[ 7 ]  FctDeclaration=extern real32_T mySqrt(real32_T u1);  FctCall=%y1 = mySqrt(%u1);  OrderingInOutPopup=None
  negprotect : Stateflow chart
  sqrt(x) : Outport
  wires:
  negprotect/1(zpVal) -> C Function Call/1
  x/1 -> negprotect/1(val)
  C Function Call/1 -> sqrt(x)/1

== system sensorMCUSlugsMKII_ren/Position and Attitude Filter/Geod2LTP1/ECEF2LTP (UEN)/From Body to Universal1/Rotation Matrix from Long//Lat ==
  note: Calculate Coefficients of DCM Row-Wise
  long lat : Inport
  11 : Fcn  Expr=cos(u[1])*cos(u[2])
  12 : Fcn  Expr=sin(u[1])*cos(u[2])
  13 : Fcn  Expr=sin(u[2])
  21 : Fcn  Expr=-sin(u[1])
  22 : Fcn  Expr=cos(u[1])
  23 : Fcn  Expr=0
  31 : Fcn  Expr=-sin(u[2])*cos(u[1])
  32 : Fcn  Expr=-sin(u[1])*sin(u[2])
  33 : Fcn  Expr=cos(u[2])
  Mux2 : Mux  Inputs=9
  DCM : Outport  InitialOutput=0
  wires:
  long lat/1 -> 21/1, 31/1, 12/1, 22/1, 32/1, 13/1, 23/1, 33/1, 11/1
  Mux2/1 -> DCM/1
  11/1 -> Mux2/1
  21/1 -> Mux2/2
  31/1 -> Mux2/3
  12/1 -> Mux2/4
  22/1 -> Mux2/5
  32/1 -> Mux2/6
  13/1 -> Mux2/7
  23/1 -> Mux2/8
  33/1 -> Mux2/9

== system sensorMCUSlugsMKII_ren/Position and Attitude Filter/Position Filter/BlendPosVel/1D Filter/Filter2 ==
  In1 : Inport
  Discrete Zero-Pole : DiscreteZeroPole  Zeros=zerosd  Poles=polesd  Gain=gaind  SampleTime=SampleTime
  Out1 : Outport
  wires:
  In1/1 -> Discrete Zero-Pole/1
  Discrete Zero-Pole/1 -> Out1/1

== system sensorMCUSlugsMKII_ren/Position and Attitude Filter/Position Filter/BlendPosVel/2 FIlter Blend/1D Filter ==
  In1 : Inport
  Data Type Conversion1 : DataTypeConversion  OutDataTypeMode=single
  Data Type Conversion2 : DataTypeConversion  OutDataTypeMode=double
  Filter2 : Subsystem  mask(DiscretizedZeroPole){Zeros=zval, Poles=pval, Gain=kval, AbsTol=auto, SampleTime=TSample, method=tustin, Wc=1}
      mask prompts: Zeros "Zeros (enter in s-main:)"; Poles "Poles (enter in s-domain:)"; Gain "Gain (enter in s-domain:)"; AbsTol "Absolute tolerance:"; SampleTime "Sample time:"; Wc "Critical Frequency (Hz):"
      mask help: Continuous mask uses c2d to transform parameters onto the Discrete Zero-Pole block inside.
      mask init: same as sensorMCUSlugsMKII_ren/Position and Attitude Filter/Attitude Complimentary Filter COG/3D Filter/Filter1
      mask StyleString: edit,edit,edit,edit,edit,popup(zoh|foh|tustin|prewarp|matched),edit
      mask CallbackString: |||||hidecrit|
      mask Display:
      | droots(zeross,poless,gainss)
      | text( 0.5, 1.0, method, 'verticalAlignment','top')
  Out1 : Outport
  wires:
  Data Type Conversion1/1 -> Out1/1
  Data Type Conversion2/1 -> Filter2/1(In1)
  In1/1 -> Data Type Conversion2/1
  Filter2/1(Out1) -> Data Type Conversion1/1

== system sensorMCUSlugsMKII_ren/Position and Attitude Filter/Position Filter/BlendPosVel/2 FIlter Blend/Tustin Lowpass,  Auto Initial Condition4 ==
  In1 : Inport
  Constant : Constant  Value=T
  Constant1 : Constant  Value=f
  Embedded MATLAB Function : Stateflow chart
  Out1 : Outport
  wires:
  Constant/1 -> Embedded MATLAB Function/2(T)
  Constant1/1 -> Embedded MATLAB Function/3(f)
  Embedded MATLAB Function/1(y) -> Out1/1
  In1/1 -> Embedded MATLAB Function/1(u)

== system sensorMCUSlugsMKII_ren/Position and Attitude Filter/Position Filter/BlendPosVel/3D Filter/Filter1 ==
  In1 : Inport
  Discrete Zero-Pole : DiscreteZeroPole  Zeros=zerosd  Poles=polesd  Gain=gaind  SampleTime=SampleTime
  Out1 : Outport
  wires:
  Discrete Zero-Pole/1 -> Out1/1
  In1/1 -> Discrete Zero-Pole/1

== system sensorMCUSlugsMKII_ren/Position and Attitude Filter/Position Filter/BlendPosVel/3D Filter/Filter2 ==
  In1 : Inport
  Discrete Zero-Pole : DiscreteZeroPole  Zeros=zerosd  Poles=polesd  Gain=gaind  SampleTime=SampleTime
  Out1 : Outport
  wires:
  In1/1 -> Discrete Zero-Pole/1
  Discrete Zero-Pole/1 -> Out1/1

== system sensorMCUSlugsMKII_ren/Position and Attitude Filter/Position Filter/BlendPosVel/3D Filter/Filter3 ==
  In1 : Inport
  Discrete Zero-Pole : DiscreteZeroPole  Zeros=zerosd  Poles=polesd  Gain=gaind  SampleTime=SampleTime
  Out1 : Outport
  wires:
  Discrete Zero-Pole/1 -> Out1/1
  In1/1 -> Discrete Zero-Pole/1

== system sensorMCUSlugsMKII_ren/Position and Attitude Filter/Position Filter/BlendPosVel/CompFiltRate/1D Filter1 ==
  In1 : Inport
  Data Type Conversion1 : DataTypeConversion  OutDataTypeMode=single
  Data Type Conversion2 : DataTypeConversion  OutDataTypeMode=double
  Filter2 : Subsystem  mask(DiscretizedZeroPole){Zeros=zval, Poles=pval, Gain=kval, AbsTol=auto, SampleTime=TSample, method=tustin, Wc=1}
      mask prompts: Zeros "Zeros (enter in s-main:)"; Poles "Poles (enter in s-domain:)"; Gain "Gain (enter in s-domain:)"; AbsTol "Absolute tolerance:"; SampleTime "Sample time:"; Wc "Critical Frequency (Hz):"
      mask help: Continuous mask uses c2d to transform parameters onto the Discrete Zero-Pole block inside.
      mask init: same as sensorMCUSlugsMKII_ren/Position and Attitude Filter/Attitude Complimentary Filter COG/3D Filter/Filter1
      mask StyleString: edit,edit,edit,edit,edit,popup(zoh|foh|tustin|prewarp|matched),edit
      mask CallbackString: |||||hidecrit|
      mask Display:
      | droots(zeross,poless,gainss)
      | text( 0.5, 1.0, method, 'verticalAlignment','top')
  Out1 : Outport
  wires:
  Data Type Conversion1/1 -> Out1/1
  Data Type Conversion2/1 -> Filter2/1(In1)
  In1/1 -> Data Type Conversion2/1
  Filter2/1(Out1) -> Data Type Conversion1/1

== system sensorMCUSlugsMKII_ren/Position and Attitude Filter/Position Filter/BlendPosVel/CompFiltRate1/1D Filter1 ==
  In1 : Inport
  Data Type Conversion1 : DataTypeConversion  OutDataTypeMode=single
  Data Type Conversion2 : DataTypeConversion  OutDataTypeMode=double
  Filter2 : Subsystem  mask(DiscretizedZeroPole){Zeros=zval, Poles=pval, Gain=kval, AbsTol=auto, SampleTime=TSample, method=tustin, Wc=1}
      mask prompts: Zeros "Zeros (enter in s-main:)"; Poles "Poles (enter in s-domain:)"; Gain "Gain (enter in s-domain:)"; AbsTol "Absolute tolerance:"; SampleTime "Sample time:"; Wc "Critical Frequency (Hz):"
      mask help: Continuous mask uses c2d to transform parameters onto the Discrete Zero-Pole block inside.
      mask init: same as sensorMCUSlugsMKII_ren/Position and Attitude Filter/Attitude Complimentary Filter COG/3D Filter/Filter1
      mask StyleString: edit,edit,edit,edit,edit,popup(zoh|foh|tustin|prewarp|matched),edit
      mask CallbackString: |||||hidecrit|
      mask Display:
      | droots(zeross,poless,gainss)
      | text( 0.5, 1.0, method, 'verticalAlignment','top')
  Out1 : Outport
  wires:
  Data Type Conversion1/1 -> Out1/1
  Data Type Conversion2/1 -> Filter2/1(In1)
  In1/1 -> Data Type Conversion2/1
  Filter2/1(Out1) -> Data Type Conversion1/1

== system sensorMCUSlugsMKII_ren/Position and Attitude Filter/Position Filter/BlendPosVel/CompRateOnly/1D Filter1 ==
  In1 : Inport
  Data Type Conversion1 : DataTypeConversion  OutDataTypeMode=single
  Data Type Conversion2 : DataTypeConversion  OutDataTypeMode=double
  Filter2 : Subsystem  mask(DiscretizedZeroPole){Zeros=zval, Poles=pval, Gain=kval, AbsTol=auto, SampleTime=TSample, method=tustin, Wc=1}
      mask prompts: Zeros "Zeros (enter in s-main:)"; Poles "Poles (enter in s-domain:)"; Gain "Gain (enter in s-domain:)"; AbsTol "Absolute tolerance:"; SampleTime "Sample time:"; Wc "Critical Frequency (Hz):"
      mask help: Continuous mask uses c2d to transform parameters onto the Discrete Zero-Pole block inside.
      mask init: same as sensorMCUSlugsMKII_ren/Position and Attitude Filter/Attitude Complimentary Filter COG/3D Filter/Filter1
      mask StyleString: edit,edit,edit,edit,edit,popup(zoh|foh|tustin|prewarp|matched),edit
      mask CallbackString: |||||hidecrit|
      mask Display:
      | droots(zeross,poless,gainss)
      | text( 0.5, 1.0, method, 'verticalAlignment','top')
  Out1 : Outport
  wires:
  Data Type Conversion1/1 -> Out1/1
  Data Type Conversion2/1 -> Filter2/1(In1)
  In1/1 -> Data Type Conversion2/1
  Filter2/1(Out1) -> Data Type Conversion1/1

== system sensorMCUSlugsMKII_ren/Sensor Data/Sensor Suite/Cube Signal Cond1/Temp Compensate Accel X/Hi Temp Compensation ==
  Raw : Inport
  Temp Raw : Inport  Port=2
  Enable : EnablePort
  Divide1 : Product  OutDataTypeMode=single  OutScaling=2^-10
  Mean Temperature for Calibration : Constant  Value=tempMean  OutDataTypeMode=single
  Sum1 : Sum  Inputs=|+-  OutDataTypeMode=single
  Sum2 : Sum  Inputs=|+-  OutDataTypeMode=single
  gains : Constant  Value=alpha  OutDataTypeMode=single
  Comp : Outport
  wires:
  Sum2/1 -> Comp/1
  Divide1/1 -> Sum2/2
  gains/1 -> Divide1/1
  Sum1/1 -> Divide1/2
  Temp Raw/1 -> Sum1/1
  Raw/1 -> Sum2/1
  Mean Temperature for Calibration/1 -> Sum1/2

== system sensorMCUSlugsMKII_ren/Sensor Data/Sensor Suite/Cube Signal Cond1/Temp Compensate Accel X/Lo Temp Compensation ==
  Raw : Inport
  Temp Raw : Inport  Port=2
  Enable : EnablePort
  Divide1 : Product  OutDataTypeMode=single  OutScaling=2^-10
  Mean Temperature for Calibration : Constant  Value=tempMean  OutDataTypeMode=single
  Sum1 : Sum  Inputs=|+-  OutDataTypeMode=single
  Sum2 : Sum  Inputs=|+-  OutDataTypeMode=single
  gains : Constant  Value=alpha  OutDataTypeMode=single
  Comp : Outport
  wires:
  Mean Temperature for Calibration/1 -> Sum1/2
  Raw/1 -> Sum2/1
  Temp Raw/1 -> Sum1/1
  Sum1/1 -> Divide1/2
  gains/1 -> Divide1/1
  Divide1/1 -> Sum2/2
  Sum2/1 -> Comp/1

== system sensorMCUSlugsMKII_ren/Sensor Data/Sensor Suite/Cube Signal Cond1/Temp Compensate Accel X/Tustin Lowpass, Auto Initial Condition1 ==
  In1 : Inport
  Constant : Constant  Value=T
  Constant1 : Constant  Value=f
  Embedded MATLAB Function : Stateflow chart
  Out1 : Outport
  wires:
  In1/1 -> Embedded MATLAB Function/1(u)
  Embedded MATLAB Function/1(y) -> Out1/1
  Constant1/1 -> Embedded MATLAB Function/3(f)
  Constant/1 -> Embedded MATLAB Function/2(T)

== system sensorMCUSlugsMKII_ren/Sensor Data/Sensor Suite/Low Pass Filtering,Temperature Compensation and Calibration1/Baro Altimeter/Compute Barometric Height ==
  Base Height (m) : Inport
  Base Pressure (Pa) : Inport  Port=2
  Baro (Pa) : Inport  Port=3
  Constant2 : Constant  Value=baseTemp/(-LapseRate)  OutDataTypeMode=single
  Constant3 : Constant  Value=9.350253e-2  OutDataTypeMode=single
  Constant4 : Constant  Value=-1.888933e-1  OutDataTypeMode=single
  Constant5 : Constant  Value=2.180313e-5  OutDataTypeMode=single
  Divide : Product  Inputs=*/  OutDataTypeMode=single  OutScaling=2^-10
  Divide{1..4} (4 alike) : Product  OutDataTypeMode=single  OutScaling=2^-10
  Length Conversion : aerolibconvert2/Length Conversion  SystemSampleTime=-1  IU=ft  OU=m
  Sum1 : Sum  Inputs=|++  OutDataTypeMode=single
  Sum2 : Sum  Inputs=|+-  OutDataTypeMode=single
  Sum3 : Sum  Inputs=3  OutDataTypeMode=single
  "Altitude, m" : Outport
  wires:
  Length Conversion/1 -> Sum1/1
  Sum2/1 -> Divide/1
  Sum1/1 -> "Altitude, m"/1
  Divide3/1 -> Length Conversion/1
  Constant2/1 -> Divide3/2
  Sum3/1 -> Divide3/1
  Constant5/1 -> Sum3/3
  Divide2/1 -> Sum3/2
  Divide1/1 -> Sum3/1
  Constant4/1 -> Divide2/2
  Constant3/1 -> Divide1/2
  Divide4/1 -> Divide1/1  "x^2"
  Divide/1 -> Divide2/1, Divide4/1, Divide4/2  "x"
  Base Pressure (Pa)/1 -> Divide/2, Sum2/2
  Base Height (m)/1 -> Sum1/2
  Baro (Pa)/1 -> Sum2/1

== system sensorMCUSlugsMKII_ren/Sensor Data/Sensor Suite/Low Pass Filtering,Temperature Compensation and Calibration1/Baro Altimeter/Enabled Subsystem ==
  In1 : Inport
  Enable : EnablePort
  Out1 : Outport  InitialOutput=baseHeight
  wires:
  In1/1 -> Out1/1

== system sensorMCUSlugsMKII_ren/Sensor Data/Sensor Suite/Low Pass Filtering,Temperature Compensation and Calibration1/Baro Altimeter/Initial Baro Bias ==
  Baro (Pa) : Inport
  Enable : EnablePort
  Data Type Conversion : DataTypeConversion  OutDataTypeMode=double
  Data Type Conversion1 : DataTypeConversion  OutDataTypeMode=single
  Low Pass8 : Subsystem  mask(DiscretizedZeroPole){Zeros=[], Poles=[-3], Gain=3, AbsTol=auto, SampleTime=.01, method=tustin, Wc=1}
      mask prompts: Zeros "Zeros (enter in s-main:)"; Poles "Poles (enter in s-domain:)"; Gain "Gain (enter in s-domain:)"; AbsTol "Absolute tolerance:"; SampleTime "Sample time:"; Wc "Critical Frequency (Hz):"
      mask help: Continuous mask uses c2d to transform parameters onto the Discrete Zero-Pole block inside.
      mask init: same as sensorMCUSlugsMKII_ren/Position and Attitude Filter/Attitude Complimentary Filter COG/3D Filter/Filter1
      mask StyleString: edit,edit,edit,edit,edit,popup(zoh|foh|tustin|prewarp|matched),edit
      mask CallbackString: |||||hidecrit|
      mask Display:
      | droots(zeross,poless,gainss)
      | text( 0.5, 1.0, method, 'verticalAlignment','top')
  Mux : Mux  Inputs=2
  Scope : Scope
      settings: SaveName=ScopeData8
  "[80k - 120k]" : Saturate  UpperLimit=120000  LowerLimit=80000
  Baro (Gnd) : Outport
  wires:
  Baro (Pa)/1 -> Data Type Conversion/1
  Low Pass8/1(Out1) -> Data Type Conversion1/1
  Data Type Conversion/1 -> Low Pass8/1(In1)
  Data Type Conversion1/1 -> Mux/2, "[80k - 120k]"/1
  Mux/1 -> Scope/1
  "[80k - 120k]"/1 -> Baro (Gnd)/1, Mux/1

== system sensorMCUSlugsMKII_ren/Sensor Data/Sensor Suite/Low Pass Filtering,Temperature Compensation and Calibration1/Baro Altimeter/Zero Out Height ==
  Base Height : Inport
  Computed Height : Inport  Port=2
  Enable : EnablePort
  Integer Delay : simulink/Discrete/Integer Delay  vinit=0  samptime=.01  NumDelays=1
  Sum : Sum  Inputs=|+-  OutDataTypeMode=single
  Height Offset : Outport
  wires:
  Computed Height/1 -> Integer Delay/1
  Sum/1 -> Height Offset/1
  Integer Delay/1 -> Sum/2
  Base Height/1 -> Sum/1

== system sensorMCUSlugsMKII_ren/Sensor Data/Sensor Suite/Low Pass Filtering,Temperature Compensation and Calibration1/Temp Compensate Accel X1/Hi Temp Compensation2 ==
  Raw : Inport
  Temp Raw : Inport  Port=2
  Enable : EnablePort
  Divide1 : Product  OutDataTypeMode=single  OutScaling=2^-10
  Mean Temperature for Calibration : Constant  Value=tempMean  OutDataTypeMode=single
  Sum1 : Sum  Inputs=|+-  OutDataTypeMode=single
  Sum2 : Sum  Inputs=|+-  OutDataTypeMode=single
  gains : Constant  Value=alpha  OutDataTypeMode=single
  Comp : Outport
  wires:
  Mean Temperature for Calibration/1 -> Sum1/2
  Raw/1 -> Sum2/1
  Temp Raw/1 -> Sum1/1
  Sum1/1 -> Divide1/2
  gains/1 -> Divide1/1
  Divide1/1 -> Sum2/2
  Sum2/1 -> Comp/1
